simulink model "TestPortF769"  (R2018b)
settings: Solver=FixedStepAuto  StartTime=0.0  StopTime=10.0  RelTol=1e-3  EnableMultiTasking=on
libraries: mbedblockslib x3, stm32f769ilib x1
settings Model: Creator=hpong  LastModifiedBy=hpong
settings OptimizationCC: StrengthReduction=on  PassReuseOutputArgsAs=Individual arguments  MaxStackSize=64  OptimizeBlockOrder=speed  OptimizationPriority=Speed  OptimizationCustomize=off
settings DebuggingCC: ParameterTunabilityLossMsg=error
settings HardwareCC: ProdBitPerPointer=32  ProdBitPerSizeT=32  ProdBitPerPtrDiffT=32  ProdLargestAtomicInteger=Long  ProdLargestAtomicFloat=Double  ProdWordSize=32  ProdHWDeviceType=ARM Compatible->ARM Cortex
settings SFSimCC: MATLABDynamicMemAlloc=off
settings RTWCC: SystemTargetFile=ert.tlc  HardwareBoard=STM32F769I-Discovery  TemplateMakefile=ert_default_tmf  GenerateReport=on  Toolchain=GNU Tools for ARM Embedded Processors  BuildConfiguration=Debug  IncludeHyperlinkInReport=on  LaunchReport=on  GenerateTraceInfo=on  GenerateTraceReport=on  GenerateTraceReportSl=on  GenerateTraceReportSf=on  GenerateTraceReportEml=on
settings CodeAppCC: ForceParamTrailComments=on  IgnoreCustomStorageClasses=off  OperatorAnnotations=on  SimulinkDataObjDesc=on  SFDataObjDesc=on  InsertBlockDesc=on

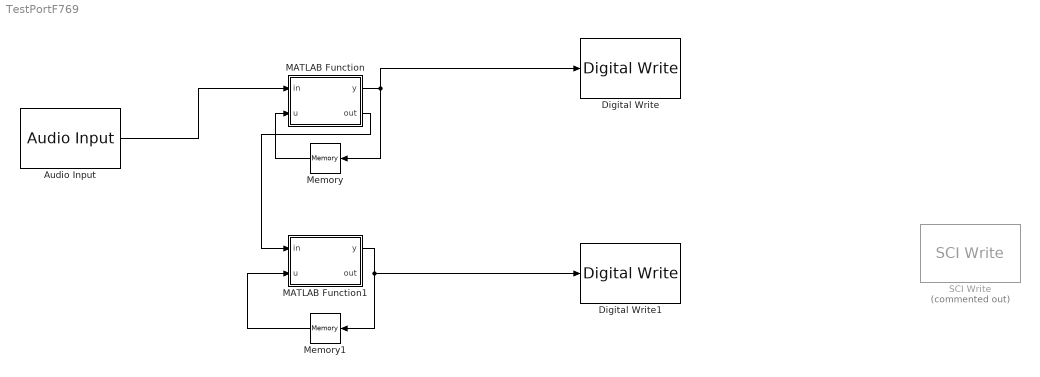
== system TestPortF769 ==
  Audio Input : stm32f769ilib/Audio Input  InputDevice=LineIn  SamplingFreq=16000  NumCh=2  FrameSize=100
      settings: SourceProductName=Embedded Coder Support Package for STMicroelectronics Discovery Boards  SourceProductBaseCode=STMICRODIS
  Digital Write : mbedblockslib/Digital Write  Pin=D7  Direction=output
      settings: SourceProductName=Simulink Coder Support Package for BBC microbit Board  SourceProductBaseCode=MICROBIT
  Digital Write1 : mbedblockslib/Digital Write  Pin=D8  Direction=output
      settings: SourceProductName=Simulink Coder Support Package for BBC microbit Board  SourceProductBaseCode=MICROBIT
  MATLAB Function : MATLAB Function  TreatAsAtomicUnit=on
  MATLAB Function1 : MATLAB Function  TreatAsAtomicUnit=on
  Memory : Memory
  Memory1 : Memory
  SCI Write : mbedblockslib/SCI Write  Commented=on  SCIModule=0  Baudrate=uint32(9600)  Parity=None  StopBits=1  HardwareFlowControl=None  ByteOrder=LittleEndian  OutputStatus=off
      settings: SourceProductName=Simulink Coder Support Package for BBC microbit Board  SourceProductBaseCode=MICROBIT
  wires:
  MATLAB Function/1(y) -> Memory/1, Digital Write/1
  Memory/1 -> MATLAB Function/2(u)
  Audio Input/1 -> MATLAB Function/1(in)
  MATLAB Function/2(out) -> MATLAB Function1/1(in)
  MATLAB Function1/1(y) -> Digital Write1/1, Memory1/1
  Memory1/1 -> MATLAB Function1/2(u)

== matlab function TestPortF769/MATLAB Function1 ==
  data: in input; u input; y output; out output
function [ y ,out ]= fcn(in,u)
pause(0.1);
% if u==1
%     y=0;
% else
%     y=1;
% end
y=1;
in = (((in+95).*4895)+25).^3;
y=0;
out = in;

== matlab function TestPortF769/MATLAB Function ==
  data: in input; u input; y output; out output
function [ y ,out ]= fcn(in,u)
if u==1
    y=0;
else
    y=1;
end

out = in;
